simulink model "ObserPlot"  (R2019a)
settings: Solver=VariableStepAuto  StartTime=0.0  StopTime=10.0  RelTol=1e-3
values from neighbouring files (symbols this model uses):
  C = C(1:3,:)    [observer.m]
  K = real(inv(R)*B'*P)    [observer.m]
  L = K_'    [observer.m]
undefined symbols (not defined in the file or in its folder): A, B
settings Model: Creator=0210s  LastModifiedBy=0210s

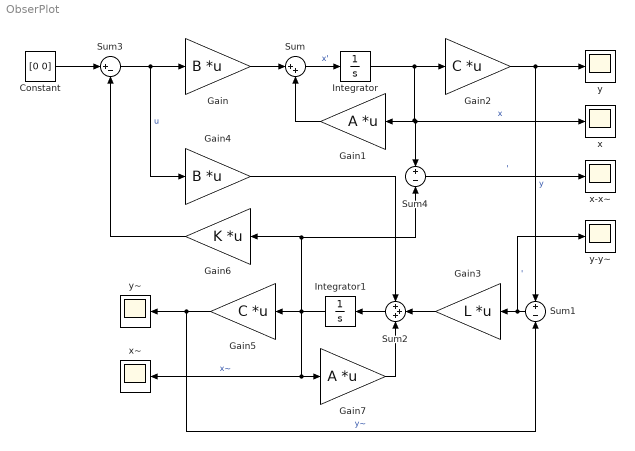
== system ObserPlot ==
  Constant : Constant  Value=[0 0]
  Gain : Gain  Gain=B  Multiplication=Matrix(K*u) (u vector)
  Gain1 : Gain  Gain=A  Multiplication=Matrix(K*u) (u vector)
  Gain2 : Gain  Gain=C  Multiplication=Matrix(K*u) (u vector)
  Gain3 : Gain  Gain=L  Multiplication=Matrix(K*u) (u vector)
  Gain4 : Gain  Gain=B  Multiplication=Matrix(K*u) (u vector)
  Gain5 : Gain  Gain=C  Multiplication=Matrix(K*u) (u vector)
  Gain6 : Gain  Gain=K  Multiplication=Matrix(K*u) (u vector)
  Gain7 : Gain  Gain=A  Multiplication=Matrix(K*u) (u vector)
  Integrator : Integrator  InitialCondition=[0.2;-0.1;0.15;-1;0.8;0]
  Integrator1 : Integrator
  Sum : Sum  Inputs=|++
  Sum1 : Sum  Inputs=+|-
  Sum2 : Sum  Inputs=+++
  Sum3 : Sum  Inputs=|+-
  Sum4 : Sum  Inputs=+|-
  x : Scope
  x-x~ : Scope
  x~ : Scope
  y : Scope
  y-y~ : Scope
  y~ : Scope
  wires:
  Sum/1 -> Integrator/1  "x'"
  Gain/1 -> Sum/1
  Integrator/1 -> Sum4/1, x/1, Gain1/1, Gain2/1  "x"
  Gain1/1 -> Sum/2
  Gain2/1 -> y/1, Sum1/1  "y"
  Sum1/1 -> y-y~/1, Gain3/1  "'"
  Gain3/1 -> Sum2/2
  Sum2/1 -> Integrator1/1
  Gain4/1 -> Sum2/1
  Gain5/1 -> y~/1, Sum1/2  "y~"
  Integrator1/1 -> Gain7/1, x~/1, Sum4/2, Gain6/1, Gain5/1  "x~"
  Gain7/1 -> Sum2/3
  Sum3/1 -> Gain4/1, Gain/1  "u"
  Gain6/1 -> Sum3/2
  Constant/1 -> Sum3/1
  Sum4/1 -> x-x~/1  "'"
